simulink model "topicFiveStructs"  (R2016a)
settings: Solver=FixedStepDiscrete  StartTime=0.0  StopTime=10.0  RelTol=1e-3
model workspace (MAT data in the model file):
  Var = 0
settings Model: Creator=LEGION  LastModifiedBy=LEGION
settings DataIOCC: SaveFormat=StructureWithTime
settings RTWCC: GenCodeOnly=on

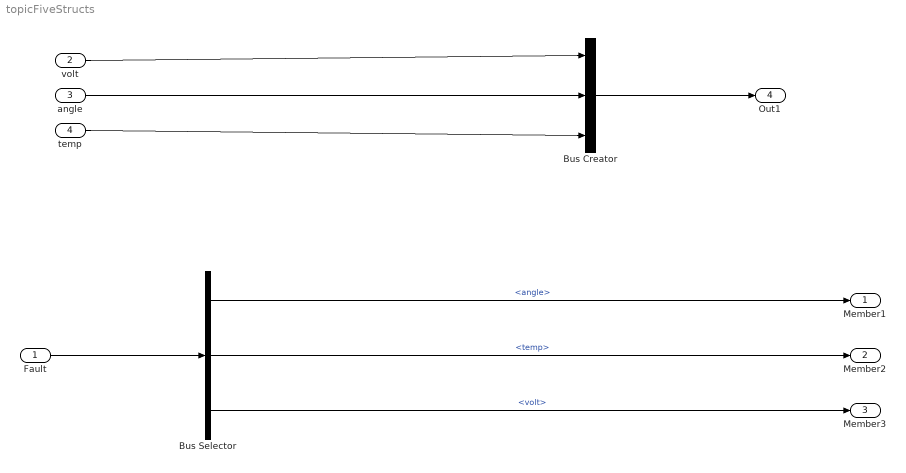
== system topicFiveStructs ==
  Fault : Inport  OutDataTypeStr=Bus: fault_t
  "volt " : Inport  Port=2
  "angle " : Inport  Port=3
  "temp " : Inport  Port=4
  Bus Creator : BusCreator  Inputs=3  OutDataTypeStr=Bus: fault_t
  Bus Selector : BusSelector  OutputSignals=angle,temp,volt
  "Member1 " : Outport
  "Member2 " : Outport  Port=2
  "Member3 " : Outport  Port=3
  Out1 : Outport  Port=4  OutDataTypeStr=Bus: fault_t
  wires:
  Fault/1 -> Bus Selector/1
  Bus Selector/1 -> "Member1 "/1  "<angle>"
  Bus Selector/2 -> "Member2 "/1  "<temp>"
  Bus Selector/3 -> "Member3 "/1  "<volt>"
  Bus Creator/1 -> Out1/1
  "volt "/1 -> Bus Creator/1
  "angle "/1 -> Bus Creator/2
  "temp "/1 -> Bus Creator/3
